simulink model "sm_trackV_roller4_artic_IdlerArm_i2u0r3_ptcld"  (R2026a)
settings: Solver=ode23t  StopTime=14  AbsTol=1e-3  EnableMultiTasking=on
PostLoadFcn:
  | set_param([bdroot '/Track FL'],'popup_sense_roller','Actuator Torque')
  | set_param([bdroot '/Track FR'],'popup_sense_roller','Actuator Torque')
  | set_param([bdroot '/Track RL'],'popup_sense_roller','Actuator Torque')
  | set_param([bdroot '/Track RR'],'popup_sense_roller','Actuator Torque')
StartFcn:
  | tic
StopFcn:
  | Elapsed_Sim_Time = toc;
  | disp(['Elapsed Sim Time = ' num2str(Elapsed_Sim_Time)]);
undefined symbols (not defined in the file): Scene, Trac, X, Y, Z
libraries: fl_lib x8, nesl_utility x6, sm_lib x4, sm_excv_chassis_lib x4, sm_trackV_lib_chain_underc_elem x4, simulink x4, sm_rollerV_lib_lower_frame_idlerArm_i2u0l3 x4, sm_rollerV_lib_terrain_contact_r5 x3
(part 2 of 2)

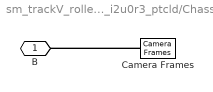
== system sm_trackV_roller4_artic_IdlerArm_i2u0r3_ptcld/Chassis ==
  Camera Frames : sm_excv_chassis_lib/Camera Frames  Camera=Trac.Chassis.Camera
  B : PMIOPort  Side=Left
  connections:
  Camera Frames/LConn1 -- B/RConn1

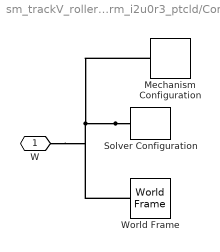
== system sm_trackV_roller4_artic_IdlerArm_i2u0r3_ptcld/Config ==
  Mechanism Configuration : sm_lib/Utilities/Mechanism Configuration  UniformGravity=Constant  GravityVector=[0 0 -9.80665]  GravityVectorUnits=m/s^2  LinearizationDelta=0.001  JointModeTransitionNonlinearIterations=2
  Solver Configuration : nesl_utility/Solver Configuration  PhysicalDomain=network_engine_domain  SubClassName=solver  LeftPortType=input  RightPortType=generic  Tones=[]  Harmonics=[]  SimulateNoise=off  Profile=off  UseLocalSampling=off  EnableSwitchedLinearOptims=on  FrequencyDomain=off  UseCCode=off  RelTol=0.001  AbsTol=1e-06  MinStep=1e-09  ToWorkspace=off  RevertToSquareIcSolve=off  NumHomotopyIterations=100  PhasorMode=off  PhasorModeNumHarmonics=1  ConsistencySolver=NEWTON_XTOL_AFTER_FTOL  CanonicalOrdering=UNORDERED  OptimizeIntermediates=UNOPTIMIZED  IndexReductionMethod=DerivativeReplacement  DoDC=off  ResidualTolerance=1e-09  ConsistencyTolSource=GLOBAL  ConsistencyAbsTol=0.001  ConsistencyRelTol=0.001  ConsistencyTolFactor=0.001  UseLocalSolver=off  LocalSolverChoice=NE_BACKWARD_EULER_ADVANCER  ResolveIndetEquations=on  FunctionEvalNumThread=1  LocalSolverSampleTime=0.001  DoFixedCost=off  MaxNonlinIter=3  MaxModeIter=2  ComputeImpulses=off  ImpulseIterations=2  LinearAlgebra=Sparse  LinearAlgebraNumThread=0  EquationFormulation=NE_TIME_EF  DelaysMemoryBudget=1024  AutomaticFiltering=on  FilteringTimeConstant=0.001  PartitionStorageMethod=AS_NEEDED  PartitionMemoryBudget=1024  PartitionMethod=FAST  MultibodyUseLocalSolver=off  MultibodyLocalSolverChoice=ODE1  MultibodyLocalSolverSampleTime=0.001
  World Frame : sm_lib/Frames and Transforms/World Frame
  W : PMIOPort  Side=Left
  connections:
  Solver Configuration/RConn1 -- Mechanism Configuration/RConn1 -- W/RConn1 -- World Frame/RConn1

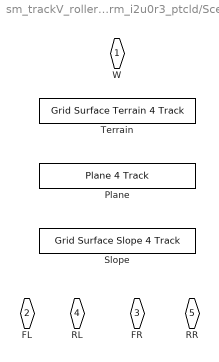
== system sm_trackV_roller4_artic_IdlerArm_i2u0r3_ptcld/Scene ==
  Plane : sm_rollerV_lib_terrain_contact_r5/Plane 4 Track  SystemSampleTime=-1  VariantControl=Plane  VariantActivationTime=update diagram  EmptyChoice=off  PassThrough=off  PassThroughVariantControl=(default)  EmptyChoiceVariantControl=(default)  AllowFlexibleInterface=on  Latency=0  AutoFrameSizeCalculation=off
  Slope : sm_rollerV_lib_terrain_contact_r5/Grid Surface Slope 4 Track  VariantControl=Slope  road_len=Scene.Slope.road_len  road_wid=Scene.Slope.road_wid*3  slope_rise=Scene.Slope.slope_rise  slope_run=Scene.Slope.slope_run  slope_x0=Scene.Slope.slope_start  slope_xres=Scene.Slope.slope_xres  surface_clr=Scene.Slope.clr  surface_opc=Scene.Slope.opc  K_Road=Scene.Contact.Terrain.K  B_Road=Scene.Contact.Terrain.B  TW_Road=Scene.Contact.Terrain.TW  F_dyn_Road=Scene.Contact.Terrain.mud  F_stat_Road=Scene.Contact.Terrain.mus  CV_Road=Scene.Contact.Terrain.CV
  Terrain : sm_rollerV_lib_terrain_contact_r5/Grid Surface Terrain 4 Track  SystemSampleTime=-1  VariantControl=Terrain  VariantActivationTime=update diagram  EmptyChoice=off  PassThrough=off  PassThroughVariantControl=(default)  EmptyChoiceVariantControl=(default)  AllowFlexibleInterface=on  Latency=0  AutoFrameSizeCalculation=off
  W : PMIOPort  Side=Right
  FL : PMIOPort  Port=2  Side=Left
  FR : PMIOPort  Port=3  Side=Left
  RL : PMIOPort  Port=4  Side=Left
  RR : PMIOPort  Port=5  Side=Left

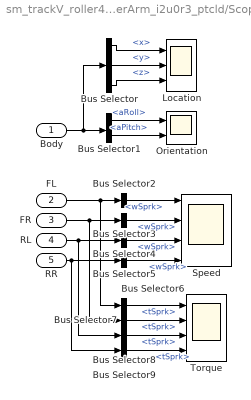
== system sm_trackV_roller4_artic_IdlerArm_i2u0r3_ptcld/Scopes ==
  Body : Inport
  FL : Inport  Port=2
  FR : Inport  Port=3
  RL : Inport  Port=4
  RR : Inport  Port=5
  Bus Selector : BusSelector  OutputSignals=x,y,z
  Bus Selector1 : BusSelector  OutputSignals=aRoll,aPitch
  Bus Selector{2..5} (4 alike) : BusSelector  OutputSignals=Underc.wSprk
  Bus Selector{6..9} (4 alike) : BusSelector  OutputSignals=Underc.tSprk
  Location : Scope  NumInputPorts=3
      settings: ActiveDisplayYMinimum=-2.438  ActiveDisplayYMaximum=13.72233
  Orientation : Scope  NumInputPorts=2
      settings: ActiveDisplayYMinimum=-0.40552  ActiveDisplayYMaximum=0.36121  DataLoggingVariableName=ScopeData2
  Speed : Scope  NumInputPorts=4
      settings: ActiveDisplayYMinimum=-0.59655  ActiveDisplayYMaximum=1.11207
  Torque : Scope  NumInputPorts=4
      settings: ActiveDisplayYMinimum=-13513.24622  ActiveDisplayYMaximum=6756.69226  DataLoggingVariableName=ScopeData2
  wires:
  Body/1 -> Bus Selector/1, Bus Selector1/1
  Bus Selector/3 -> Location/3  "<z>"
  RL/1 -> Bus Selector8/1, Bus Selector4/1
  Bus Selector1/1 -> Orientation/1  "<aRoll>"
  Bus Selector/2 -> Location/2  "<y>"
  Bus Selector/1 -> Location/1  "<x>"
  Bus Selector1/2 -> Orientation/2  "<aPitch>"
  RR/1 -> Bus Selector9/1, Bus Selector5/1
  FR/1 -> Bus Selector7/1, Bus Selector3/1
  FL/1 -> Bus Selector6/1, Bus Selector2/1
  Bus Selector2/1 -> Speed/1  "<wSprk>"
  Bus Selector3/1 -> Speed/2  "<wSprk>"
  Bus Selector4/1 -> Speed/3  "<wSprk>"
  Bus Selector5/1 -> Speed/4  "<wSprk>"
  Bus Selector6/1 -> Torque/1  "<tSprk>"
  Bus Selector7/1 -> Torque/2  "<tSprk>"
  Bus Selector8/1 -> Torque/3  "<tSprk>"
  Bus Selector9/1 -> Torque/4  "<tSprk>"

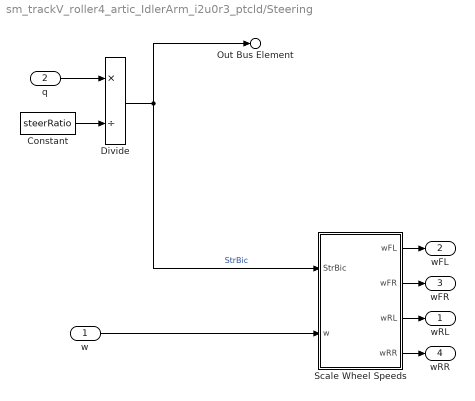
== system sm_trackV_roller4_artic_IdlerArm_i2u0r3_ptcld/Steering ==
  w : Inport
  q : Inport  Port=2
  Constant : Constant  Value=steerRatio
  Divide : Product  Inputs=*/
  Scale Wheel Speeds : Subsystem
  wRL : Outport
  wFL : Outport  Port=2
  wFR : Outport  Port=3
  wRR : Outport  Port=4
  Out Bus Element : Outport  Port=5  PortName=m  Element=SteerBicycle
  wires:
  Scale Wheel Speeds/4(wRR) -> wRR/1
  Scale Wheel Speeds/3(wRL) -> wRL/1
  Scale Wheel Speeds/2(wFR) -> wFR/1
  Scale Wheel Speeds/1(wFL) -> wFL/1
  w/1 -> Scale Wheel Speeds/2(w)
  Divide/1 -> Scale Wheel Speeds/1(StrBic), Out Bus Element/1  "StrBic"
  Constant/1 -> Divide/2
  q/1 -> Divide/1

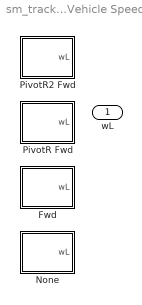
== system sm_trackV_roller4_artic_IdlerArm_i2u0r3_ptcld/Vehicle Speed ==
  Fwd : Subsystem  VariantControl=Fwd
  None : Subsystem  VariantControl=None
  PivotR Fwd : Subsystem  VariantControl=PivotR_Fwd
  PivotR2 Fwd : Subsystem  VariantControl=PivotR2_Fwd
  wL : Outport

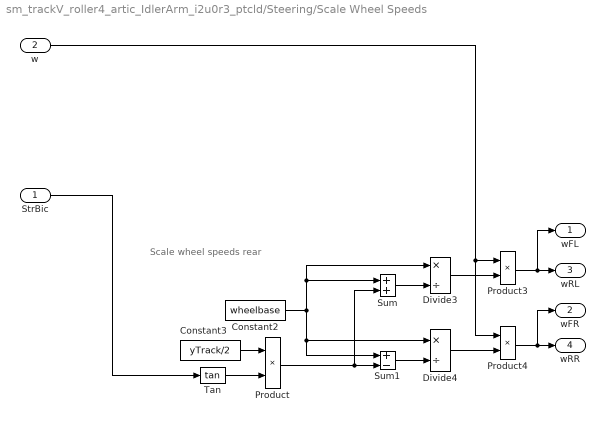
== system sm_trackV_roller4_artic_IdlerArm_i2u0r3_ptcld/Steering/Scale Wheel Speeds ==
  note: Scale wheel speeds rear
  StrBic : Inport
  w : Inport  Port=2
  Constant2 : Constant  Value=wheelbase
  Constant3 : Constant  Value=yTrack/2
  Divide3 : Product  Inputs=*/
  Divide4 : Product  Inputs=*/
  Product : Product
  Product3 : Product
  Product4 : Product
  Sum : Sum
  Sum1 : Sum  Inputs=+-
  Tan : Trigonometry  Operator=tan
  wFL : Outport
  wFR : Outport  Port=2
  wRL : Outport  Port=3
  wRR : Outport  Port=4
  wires:
  Divide3/1 -> Product3/2
  Divide4/1 -> Product4/2
  Product4/1 -> wFR/1, wRR/1
  Product/1 -> Sum1/2, Sum/2
  Tan/1 -> Product/2
  Sum1/1 -> Divide4/2
  StrBic/1 -> Tan/1
  Product3/1 -> wFL/1, wRL/1
  w/1 -> Product4/1, Product3/1
  Sum/1 -> Divide3/2
  Constant2/1 -> Divide4/1, Sum1/1, Sum/1, Divide3/1
  Constant3/1 -> Product/1

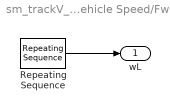
== system sm_trackV_roller4_artic_IdlerArm_i2u0r3_ptcld/Vehicle Speed/Fwd ==
  Repeating Sequence : simulink/Sources/Repeating Sequence  rep_seq_t=[0 2 2.01 60]  rep_seq_y=[0 0 3 3]
  wL : Outport
  wires:
  Repeating Sequence/1 -> wL/1

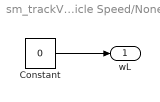
== system sm_trackV_roller4_artic_IdlerArm_i2u0r3_ptcld/Vehicle Speed/None ==
  Constant : Constant  Value=0
  wL : Outport
  wires:
  Constant/1 -> wL/1

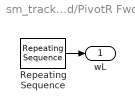
== system sm_trackV_roller4_artic_IdlerArm_i2u0r3_ptcld/Vehicle Speed/PivotR Fwd ==
  Repeating Sequence : simulink/Sources/Repeating Sequence  rep_seq_t=[0 2 2.01 40]  rep_seq_y=[0 0 3 3]
  wL : Outport
  wires:
  Repeating Sequence/1 -> wL/1

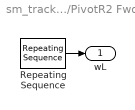
== system sm_trackV_roller4_artic_IdlerArm_i2u0r3_ptcld/Vehicle Speed/PivotR2 Fwd ==
  Repeating Sequence : simulink/Sources/Repeating Sequence  rep_seq_t=[0 2 2.01 40]  rep_seq_y=[0 0 3 3]
  wL : Outport
  wires:
  Repeating Sequence/1 -> wL/1
